simulink model "BicyclePeterCorkePathFollow"  (R2021a)
settings: Solver=VariableStepAuto  StartTime=0.0  StopTime=1000  RelTol=1e-3
values from neighbouring files (symbols this model uses):
  accelLim = 1    [BicyclePeterCorkeP2PSetup.m]    (also in BicyclePeterCorkeSetup.m)
  initCoord = [8 5 pi/2]    [BicyclePeterCorkeP2PSetup.m]    (also in BicyclePeterCorkeSetup.m)
  speedLim = 1    [BicyclePeterCorkeP2PSetup.m]    (also in BicyclePeterCorkeSetup.m)
  steerLim = 1    [BicyclePeterCorkeP2PSetup.m]    (also in BicyclePeterCorkeSetup.m)
  wheelBase = 1    [BicyclePeterCorkeP2PSetup.m]    (also in BicyclePeterCorkeSetup.m)
undefined symbols (not defined in the file or in its folder): path
libraries: robotalgslib x1, simulink x1
settings Model: Creator=User  LastModifiedBy=User

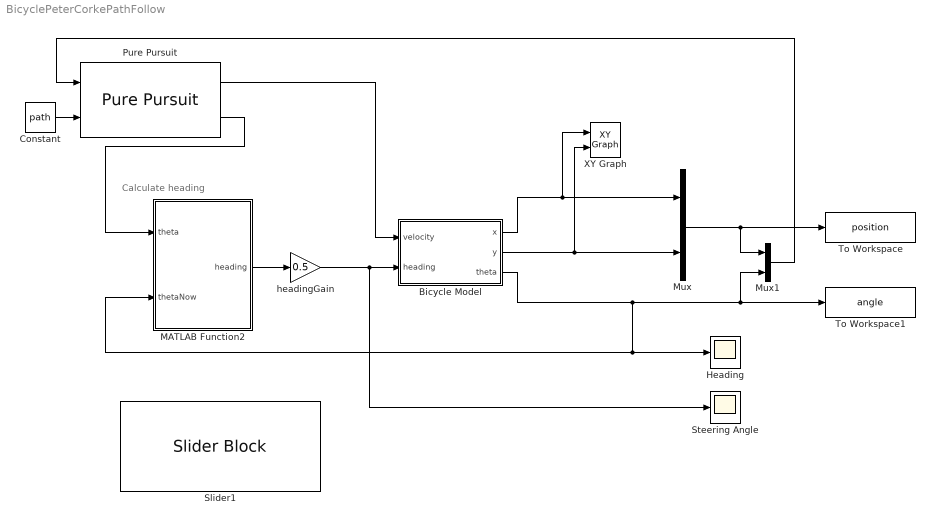
== system BicyclePeterCorkePathFollow ==
  note: Calculate heading
  Bicycle Model : Subsystem
  Constant : Constant  Value=path
  Heading : Scope
  MATLAB Function2 : MATLAB Function  TreatAsAtomicUnit=on
  Mux : Mux  Inputs=2
  Mux1 : Mux  Inputs=2
  Pure Pursuit : robotalgslib/Pure Pursuit  DesiredLinearVelocity=1  MaxAngularVelocity=1.0  LookaheadDistance=5  TargetDirPort=off  SimulateUsing=Code generation
  Slider1 : SliderBlock  ScaleMax=5
  Steering Angle : Scope
  To Workspace : ToWorkspace  VariableName=position  SaveFormat=Timeseries  SampleTime=-1
  To Workspace1 : ToWorkspace  VariableName=angle  SaveFormat=Timeseries  SampleTime=-1
  XY Graph : simulink/Sinks/XY Graph  xmin=-2  xmax=10  ymin=-2  ymax=10  st=-1
  headingGain : Gain  Gain=0.5
  wires:
  Bicycle Model/2(y) -> Mux/2, XY Graph/2
  Bicycle Model/1(x) -> Mux/1, XY Graph/1
  Pure Pursuit/2 -> MATLAB Function2/1(theta)
  Mux/1 -> Mux1/1, To Workspace/1
  MATLAB Function2/1(heading) -> headingGain/1
  Bicycle Model/3(theta) -> Mux1/2, To Workspace1/1, MATLAB Function2/2(thetaNow), Heading/1
  headingGain/1 -> Steering Angle/1, Bicycle Model/2(heading)
  Pure Pursuit/1 -> Bicycle Model/1(velocity)
  Mux1/1 -> Pure Pursuit/1
  Constant/1 -> Pure Pursuit/2

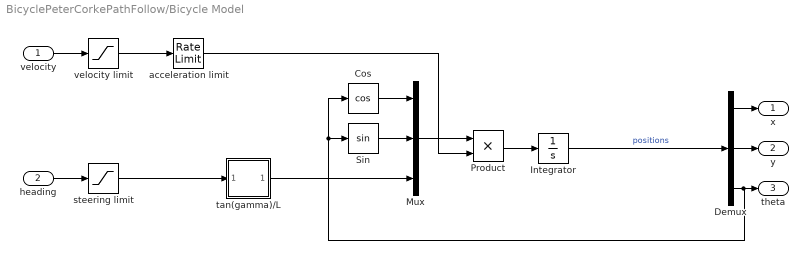
== system BicyclePeterCorkePathFollow/Bicycle Model ==
  velocity : Inport
  heading : Inport  Port=2
  Cos : Trigonometry  Operator=cos
  Demux : Demux  Outputs=3
  Integrator : Integrator  InitialCondition=initCoord
  Mux : Mux  Inputs=3
  Product : Product
  Sin : Trigonometry
  acceleration limit : RateLimiter  RisingSlewLimit=accelLim  FallingSlewLimit=-accelLim  SampleTimeMode=inherited
  steering limit : Saturate  UpperLimit=steerLim  LowerLimit=-steerLim
  tan(gamma)/L : Subsystem
  velocity limit : Saturate  UpperLimit=speedLim  LowerLimit=-speedLim
  x : Outport
  y : Outport  Port=2
  theta : Outport  Port=3
  wires:
  velocity/1 -> velocity limit/1
  velocity limit/1 -> acceleration limit/1
  heading/1 -> steering limit/1
  steering limit/1 -> tan(gamma)/L/1(In1)
  tan(gamma)/L/1(Out1) -> Mux/3
  Mux/1 -> Product/1
  acceleration limit/1 -> Product/2
  Product/1 -> Integrator/1
  Integrator/1 -> Demux/1  "positions"
  Demux/3 -> Cos/1, Sin/1, theta/1
  Demux/1 -> x/1
  Demux/2 -> y/1
  Cos/1 -> Mux/1
  Sin/1 -> Mux/2

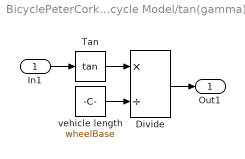
== system BicyclePeterCorkePathFollow/Bicycle Model/tan(gamma)//L ==
  In1 : Inport
  Divide : Product  Inputs=*/
  Tan : Trigonometry  Operator=tan
  vehicle length : Constant  Value=wheelBase
  Out1 : Outport
  wires:
  Tan/1 -> Divide/1
  vehicle length/1 -> Divide/2
  In1/1 -> Tan/1
  Divide/1 -> Out1/1

== matlab function BicyclePeterCorkePathFollow/MATLAB Function2 ==
  data: theta input; heading output; thetaNow input
function heading = gammaGoal(theta, thetaNow)

heading = angdiff(thetaNow, theta);
